simulink model "rx_cpm"  (R2014b)
settings: Solver=ode45  StartTime=0.0  StopTime=inf  RelTol=1e-3
libraries: dsparch4 x2, siglabs_lib x2, commsdrhw_v2 x1
settings Model: Creator=Ben  LastModifiedBy=echiu

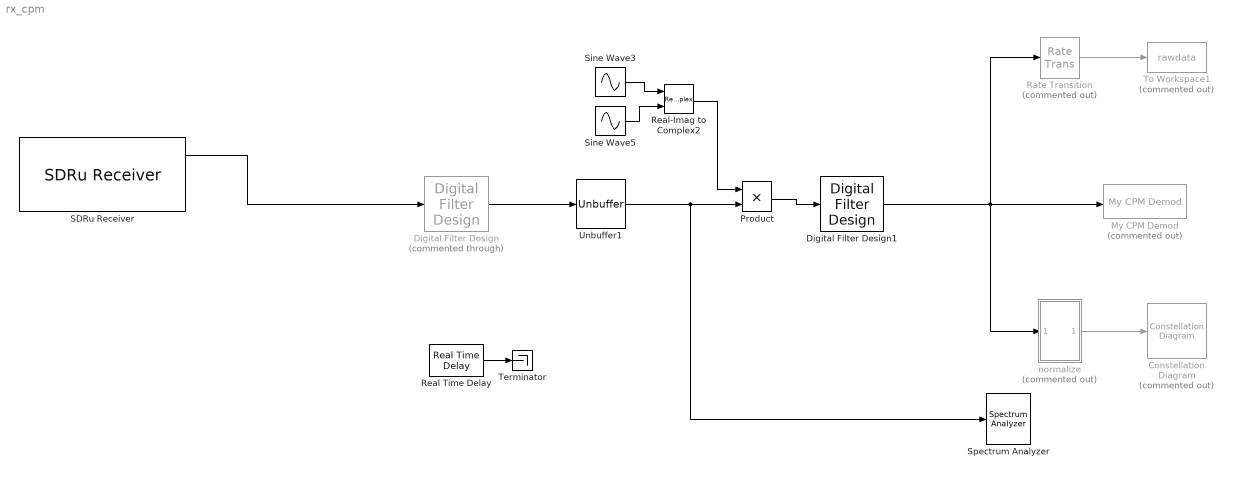
== system rx_cpm ==
  Constellation Diagram : ConstellationDiagram  Commented=on
  Digital Filter Design : dsparch4/Digital Filter Design  Commented=through  mwdsp_browser_bugfix_var=off
  Digital Filter Design1 : dsparch4/Digital Filter Design  mwdsp_browser_bugfix_var=off
  My CPM Demod : siglabs_lib/My CPM Demod  Commented=on  SampsPerSym=10  RotationsPerSym=1  PatternVectorDialog=[0]  PatternVectorRepeatDialog=2
  Product : Product
  Rate Transition : RateTransition  Commented=on  Deterministic=off  OutPortSampleTime=1/125000
  Real Time Delay : siglabs_lib/Real Time Delay  TimeDelay=2
  Real-Imag to Complex2 : RealImagToComplex
  SDRu Receiver : commsdrhw_v2/SDRu Receiver  rxtx=rx  platform=N200/N210/USRP2  USRP2_IP='192.168.10.2'  USRP_IP_X300='192.168.10.2'  USRP_IP_X310='192.168.10.2'  USRP_serialNumB200=''  USRP_serialNumB210=''  centerFrequency=915E6  centerFrequencySrc=Dialog  loOffset=0  loOffsetSrc=Dialog  masterClkRateB200=32e6  masterClkRateB210=32e6  masterClkRateX300=200e6  masterClkRateX310=200e6  masterClkRateParam=100e6  gain=32  gainSrc=Dialog  decimInterp=512  decimInterpSrc=Dialog  USRP2_IP_NUM=[49 57 50 46 49 54 56 46 49 48 46 50]  frameLength=1024  outputDatatype=double  overrunUnderrunPort=off  sampleTime=512/1E8  HOST_DATA_PORT=0  HOST_CONTROL_PORT=0  USRP2_DATA_PORT=0  USRP2_CONTROL_PORT=0  bufferMode=Continuous streaming  EnableBurstMode=off  NumFramesInBurst=1  USRP_ID='192.168.10.2'
  Sine Wave3 : Sin  Frequency=2*pi*20000  Phase=1.5*pi  SampleTime=512/1E8
  Sine Wave5 : Sin  Frequency=2*pi*20000  SampleTime=512/1E8
  Spectrum Analyzer : SpectrumAnalyzer
  Terminator : Terminator
  To Workspace1 : ToWorkspace  Commented=on  VariableName=rawdata  SampleTime=-1
      settings: Save2DSignal=2-D array (concatenate along first dimension)
  Unbuffer1 : Unbuffer  SampleBasedProcessing=Same as frame based
  normalize : Subsystem  Commented=on
  wires:
  Digital Filter Design/1 -> Unbuffer1/1
  SDRu Receiver/1 -> Digital Filter Design/1
  Real-Imag to Complex2/1 -> Product/1
  Unbuffer1/1 -> Spectrum Analyzer/1, Product/2
  Product/1 -> Digital Filter Design1/1
  Sine Wave5/1 -> Real-Imag to Complex2/2
  Sine Wave3/1 -> Real-Imag to Complex2/1
  normalize/1(Out1) -> Constellation Diagram/1
  Digital Filter Design1/1 -> My CPM Demod/1, normalize/1(In1), Rate Transition/1
  Rate Transition/1 -> To Workspace1/1
  Real Time Delay/1 -> Terminator/1

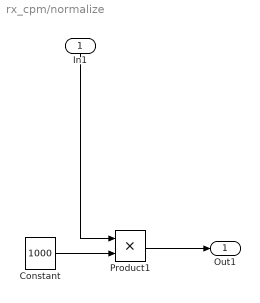
== system rx_cpm/normalize ==
  In1 : Inport
  Constant : Constant  Value=1000
  Product1 : Product
  Out1 : Outport
  wires:
  Product1/1 -> Out1/1
  In1/1 -> Product1/1
  Constant/1 -> Product1/2
